simulink model "model"  (R2024b)
settings: Solver=ode4  StartTime=0.0  StopTime=tf  FixedStep=dt  RelTol=1e-3
values from neighbouring files (symbols this model uses):
  Controls_Matrix = [0,    XDE,   XDTH,      0 ... (first row only)    [aircraft_data_reader.m]
  dA = controls(1)    [compare_nonlinear_linear_approximate_simulator.m]
  dE = controls(2)    [compare_nonlinear_linear_approximate_simulator.m]
  dR = controls(4)    [compare_nonlinear_linear_approximate_simulator.m]
  dTH = controls(3)    [compare_nonlinear_linear_approximate_simulator.m]
  g = aircraft_data(52)    [aircraft_data_reader.m]
  Ixx = aircraft_data(53)    [aircraft_data_reader.m]
  Iyy = aircraft_data(54)    [aircraft_data_reader.m]
  Izz = aircraft_data(55)    [aircraft_data_reader.m]
  m = aircraft_data(51)    [aircraft_data_reader.m]
  mg0 = m*g * [ sin(s0(8)) ; -cos(s0(8))*sin(s0(7)) ; -cos(s0(8))*cos(s0(7)) ]    [aircraft_data_reader.m]
  p = states(4)    [Fdot.m]
  phi = states(7)    [Fdot.m]
  psi = states(9)    [Fdot.m]
  q = states(5)    [Fdot.m]
  r = states(6)    [Fdot.m]
  s0 = aircraft_data(4:15)    [aircraft_data_reader.m]
  States_Matrix = [Xu,   0,   Xw,    0,   0,   0,    0 ... (first row only)    [aircraft_data_reader.m]
  theta = states(8)    [Fdot.m]
  v = states(2)    [Fdot.m]
  w = states(3)    [Fdot.m]
  wdot = K4(3)    [RK4.m]
  x = states(10)    [Fdot.m]
  y = states(11)    [Fdot.m]
  z = states(12)    [Fdot.m]
undefined symbols (not defined in the file or in its folder): alpha, beta, d_a, d_e, d_r, d_th, initial_states_bus
libraries: simulink_extras x8, dspsigops x3, shared6dof x1, aerolibasang x1
settings Model: Creator=ahmed  LastModifiedBy=ahmed
settings DebuggingCC: SignalInfNanChecking=warning  CheckMatrixSingularityMsg=warning  SignalLabelMismatchMsg=warning  StateNameClashWarn=warning

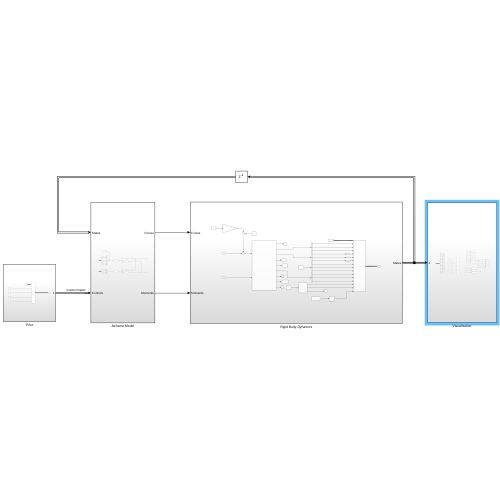
[thumbnail: Simulink's stored preview of the top-level diagram]
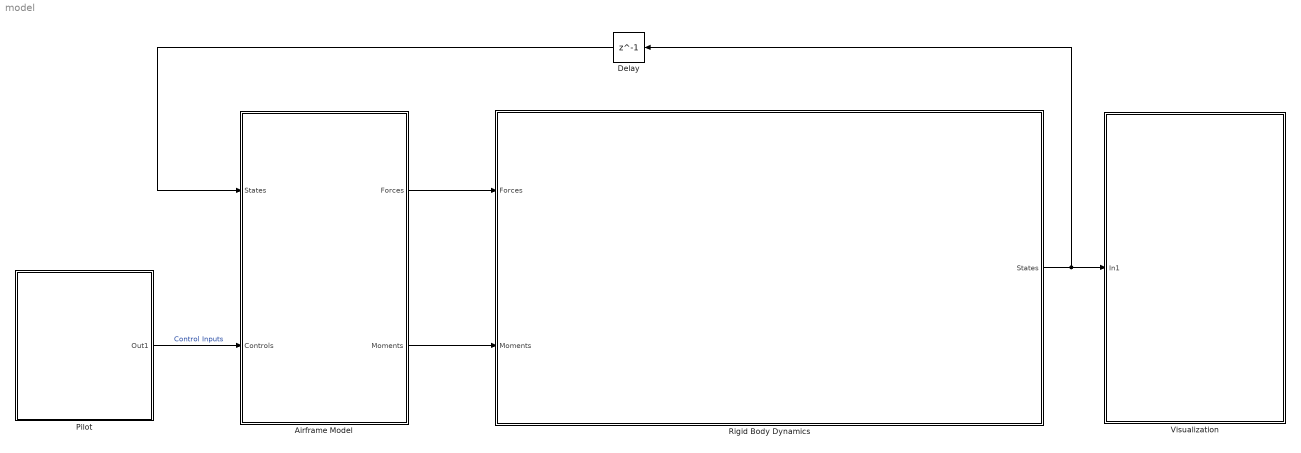
== system model ==
  Airframe Model : Subsystem
  Delay : Delay  DelayLength=1  InitialCondition=initial_states_bus
  Pilot : Subsystem
  Rigid Body Dynamics : Subsystem
  Visualization : Subsystem
  wires:
  Pilot/1(Out1) -> Airframe Model/2(Controls)  "Control Inputs"
  Airframe Model/1(Forces) -> Rigid Body Dynamics/1(Forces)
  Airframe Model/2(Moments) -> Rigid Body Dynamics/2(Moments)
  Rigid Body Dynamics/1(States) -> Visualization/1(In1), Delay/1
  Delay/1 -> Airframe Model/1(States)

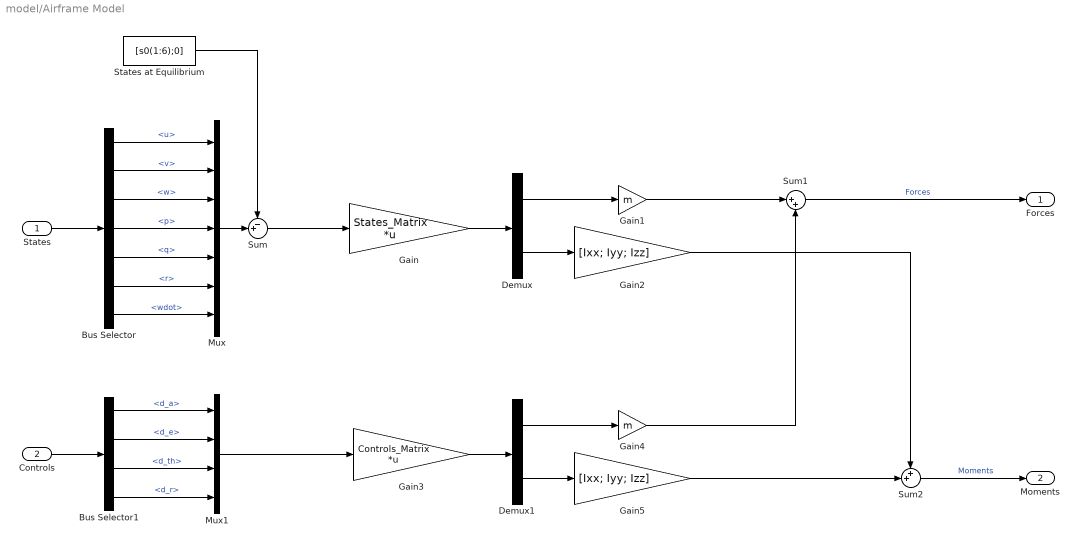
== system model/Airframe Model ==
  States : Inport  OutDataTypeStr=Bus: States_bus_T
  Controls : Inport  Port=2  OutDataTypeStr=Bus: Controls_bus_T
  Bus Selector : BusSelector  OutputSignals=u,v,w,p,q,r,wdot
  Bus Selector1 : BusSelector  OutputSignals=d_a,d_e,d_th,d_r
  Demux : Demux  Outputs=2
  Demux1 : Demux  Outputs=2
  Gain : Gain  Gain=States_Matrix  Multiplication=Matrix(K*u)
  Gain1 : Gain  Gain=m
  Gain2 : Gain  Gain=[Ixx; Iyy; Izz]
  Gain3 : Gain  Gain=Controls_Matrix  Multiplication=Matrix(K*u)
  Gain4 : Gain  Gain=m
  Gain5 : Gain  Gain=[Ixx; Iyy; Izz]
  Mux : Mux  Inputs=7
  Mux1 : Mux
  States at Equilibrium : Constant  Value=[s0(1:6);0]
  Sum : Sum  Inputs=-+|
  Sum1 : Sum  Inputs=|++
  Sum2 : Sum  Inputs=++|
  Forces : Outport
  Moments : Outport  Port=2
  wires:
  Sum1/1 -> Forces/1  "Forces"
  Sum2/1 -> Moments/1  "Moments"
  States/1 -> Bus Selector/1
  Bus Selector/2 -> Mux/2  "<v>"
  Bus Selector/1 -> Mux/1  "<u>"
  Bus Selector/3 -> Mux/3  "<w>"
  Bus Selector/4 -> Mux/4  "<p>"
  Bus Selector/5 -> Mux/5  "<q>"
  Bus Selector/6 -> Mux/6  "<r>"
  Bus Selector/7 -> Mux/7  "<wdot>"
  Mux/1 -> Sum/2
  States at Equilibrium/1 -> Sum/1
  Sum/1 -> Gain/1
  Gain/1 -> Demux/1
  Demux/1 -> Gain1/1
  Demux/2 -> Gain2/1
  Gain1/1 -> Sum1/1
  Gain2/1 -> Sum2/1
  Demux1/2 -> Gain5/1
  Gain3/1 -> Demux1/1
  Controls/1 -> Bus Selector1/1
  Bus Selector1/3 -> Mux1/3  "<d_th>"
  Bus Selector1/2 -> Mux1/2  "<d_e>"
  Bus Selector1/1 -> Mux1/1  "<d_a>"
  Bus Selector1/4 -> Mux1/4  "<d_r>"
  Mux1/1 -> Gain3/1
  Gain5/1 -> Sum2/2
  Demux1/1 -> Gain4/1
  Gain4/1 -> Sum1/2

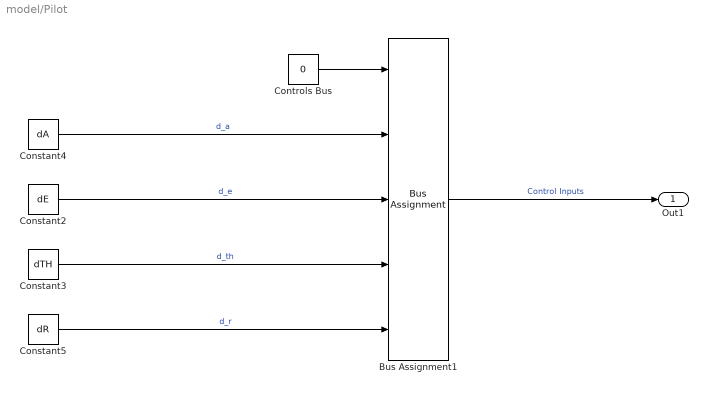
== system model/Pilot ==
  Bus Assignment1 : BusAssignment  AssignedSignals=d_a,d_e,d_th,d_r
  Constant2 : Constant  Value=dE
  Constant3 : Constant  Value=dTH
  Constant4 : Constant  Value=dA
  Constant5 : Constant  Value=dR
  Controls Bus : Constant  Value=0  OutDataTypeStr=Bus: Controls_bus_T
  Out1 : Outport
  wires:
  Constant2/1 -> Bus Assignment1/3  "d_e"
  Constant4/1 -> Bus Assignment1/2  "d_a"
  Constant5/1 -> Bus Assignment1/5  "d_r"
  Constant3/1 -> Bus Assignment1/4  "d_th"
  Controls Bus/1 -> Bus Assignment1/1
  Bus Assignment1/1 -> Out1/1  "Control Inputs"

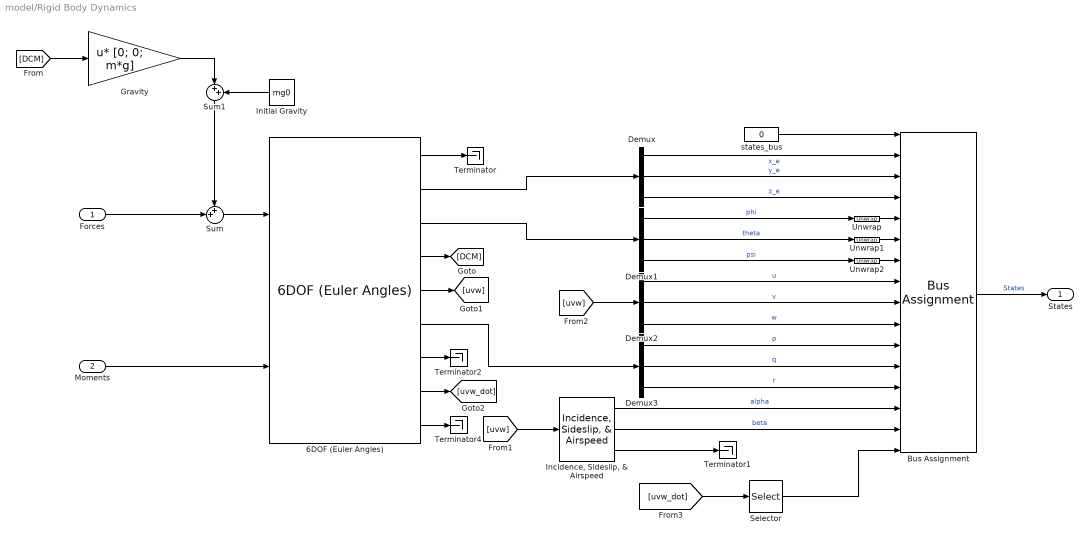
== system model/Rigid Body Dynamics ==
  Forces : Inport
  Moments : Inport  Port=2
  6DOF (Euler Angles) : shared6dof/6DOF (Euler Angles)  units=English (Velocity in ft/s)  mtype=Fixed  rep=Euler Angles  xme_0=s0(10:12)  Vm_0=s0(1:3)  eul_0=s0(7:9)  pm_0=s0(4:6)  mass_0=m  mass_e=0.5  mass_f=2.0  inertia=I  inertia_e=eye(3)  inertia_f=2*eye(3)  k_quat=1.0  vre_flag=on  abi_flag=on  aMode=0  xme_statename=''  Vm_statename=''  eul_statename=''  quat_statename=''  pm_statename=''  mass_statename=''
  Bus Assignment : BusAssignment  AssignedSignals=x,y,z,phi,theta,psi,u,v,w,p,q,r,alpha,beta,wdot
  Demux{,1..3} (4 alike) : Demux  Outputs=3
  Gravity : Gain  Gain=[0; 0; m*g]  Multiplication=Matrix(u*K)
  "Incidence, Sideslip, & Airspeed" : aerolibasang/Incidence, Sideslip, & Airspeed
  Initial Gravity : Constant  Value=mg0
  Selector : Selector  InputPortWidth=3  IndexOptions=Index vector (dialog)  Indices=3  OutputSizes=1
  Sum : Sum  Inputs=++|
  Sum1 : Sum  Inputs=|++
  Terminator{,1..2,4} (4 alike) : Terminator
  Unwrap : dspsigops/Unwrap  tol=pi  running=off
  Unwrap1 : dspsigops/Unwrap  tol=pi  running=off
  Unwrap2 : dspsigops/Unwrap  tol=pi  running=off
  states_bus : Constant  Value=0  OutDataTypeStr=Bus: States_bus_T
  States : Outport  OutDataTypeStr=Bus: States_bus_T
  wires:
  Bus Assignment/1 -> States/1  "States"
  Demux1/2 -> Unwrap1/1  "theta"
  Demux3/2 -> Bus Assignment/12  "q"
  6DOF (Euler Angles)/7 -> Terminator2/1
  6DOF (Euler Angles)/1 -> Terminator/1
  6DOF (Euler Angles)/3 -> Demux1/1
  states_bus/1 -> Bus Assignment/1
  Forces/1 -> Sum/2
  6DOF (Euler Angles)/6 -> Demux3/1
  6DOF (Euler Angles)/8 -> [uvw_dot]
  Demux2/2 -> Bus Assignment/9  "v"
  Demux1/3 -> Unwrap2/1  "psi"
  Demux3/3 -> Bus Assignment/13  "r"
  Demux2/1 -> Bus Assignment/8  "u"
  Demux2/3 -> Bus Assignment/10  "w"
  6DOF (Euler Angles)/2 -> Demux/1
  Demux/3 -> Bus Assignment/4  "z_e"
  Demux1/1 -> Unwrap/1  "phi"
  Demux/2 -> Bus Assignment/3  "y_e"
  Demux/1 -> Bus Assignment/2  "x_e"
  6DOF (Euler Angles)/9 -> Terminator4/1
  Demux3/1 -> Bus Assignment/11  "p"
  6DOF (Euler Angles)/4 -> [DCM]
  Unwrap/1 -> Bus Assignment/5
  Unwrap1/1 -> Bus Assignment/6
  Unwrap2/1 -> Bus Assignment/7
  [DCM] -> Gravity/1
  Gravity/1 -> Sum1/1
  Initial Gravity/1 -> Sum1/2
  Sum1/1 -> Sum/1
  Sum/1 -> 6DOF (Euler Angles)/1
  6DOF (Euler Angles)/5 -> [uvw]
  [uvw] -> "Incidence, Sideslip, & Airspeed"/1
  "Incidence, Sideslip, & Airspeed"/3 -> Terminator1/1
  "Incidence, Sideslip, & Airspeed"/2 -> Bus Assignment/15  "beta"
  "Incidence, Sideslip, & Airspeed"/1 -> Bus Assignment/14  "alpha"
  [uvw] -> Demux2/1
  Moments/1 -> 6DOF (Euler Angles)/2
  [uvw_dot] -> Selector/1
  Selector/1 -> Bus Assignment/16

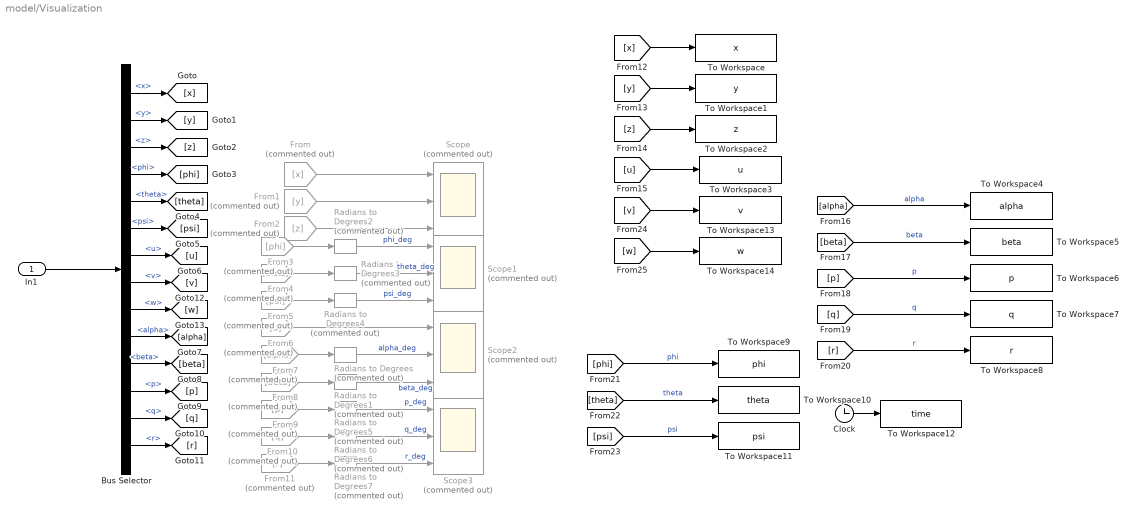
== system model/Visualization ==
  In1 : Inport
  Bus Selector : BusSelector  OutputSignals=x,y,z,phi,theta,psi,u,v,w,alpha,beta,p,q,r
  Clock : Clock
  From : From  Commented=on  GotoTag=x
  From1 : From  Commented=on  GotoTag=y
  From10 : From  Commented=on  GotoTag=q
  From11 : From  Commented=on  GotoTag=r
  From2 : From  Commented=on  GotoTag=z
  From3 : From  Commented=on  GotoTag=phi
  From4 : From  Commented=on  GotoTag=theta
  From5 : From  Commented=on  GotoTag=psi
  From6 : From  Commented=on  GotoTag=u
  From7 : From  Commented=on  GotoTag=alpha
  From8 : From  Commented=on  GotoTag=beta
  From9 : From  Commented=on  GotoTag=p
  Radians to Degrees{,1..7} (8 alike) : simulink_extras/Transformations/Radians to Degrees  Commented=on
  Scope{,1..3} (4 alike) : Scope  Commented=on  NumInputPorts=3
  To Workspace : ToWorkspace  VariableName=x  SaveFormat=Timeseries  SampleTime=-1
  To Workspace1 : ToWorkspace  VariableName=y  SaveFormat=Timeseries  SampleTime=-1
  To Workspace10 : ToWorkspace  VariableName=theta  SaveFormat=Timeseries  SampleTime=-1
  To Workspace11 : ToWorkspace  VariableName=psi  SaveFormat=Timeseries  SampleTime=-1
  To Workspace12 : ToWorkspace  VariableName=time  SaveFormat=Timeseries  SampleTime=-1
  To Workspace13 : ToWorkspace  VariableName=v  SaveFormat=Timeseries  SampleTime=-1
  To Workspace14 : ToWorkspace  VariableName=w  SaveFormat=Timeseries  SampleTime=-1
  To Workspace2 : ToWorkspace  VariableName=z  SaveFormat=Timeseries  SampleTime=-1
  To Workspace3 : ToWorkspace  VariableName=u  SaveFormat=Timeseries  SampleTime=-1
  To Workspace4 : ToWorkspace  VariableName=alpha  SaveFormat=Timeseries  SampleTime=-1
  To Workspace5 : ToWorkspace  VariableName=beta  SaveFormat=Timeseries  SampleTime=-1
  To Workspace6 : ToWorkspace  VariableName=p  SaveFormat=Timeseries  SampleTime=-1
  To Workspace7 : ToWorkspace  VariableName=q  SaveFormat=Timeseries  SampleTime=-1
  To Workspace8 : ToWorkspace  VariableName=r  SaveFormat=Timeseries  SampleTime=-1
  To Workspace9 : ToWorkspace  VariableName=phi  SaveFormat=Timeseries  SampleTime=-1
  wires:
  Bus Selector/6 -> [psi]  "<psi>"
  Bus Selector/1 -> [x]  "<x>"
  Bus Selector/7 -> [u]  "<u>"
  Bus Selector/4 -> [phi]  "<phi>"
  Bus Selector/10 -> [alpha]  "<alpha>"
  Bus Selector/14 -> [r]  "<r>"
  Bus Selector/11 -> [beta]  "<beta>"
  Bus Selector/5 -> [theta]  "<theta>"
  Bus Selector/13 -> [q]  "<q>"
  Bus Selector/12 -> [p]  "<p>"
  Bus Selector/2 -> [y]  "<y>"
  Bus Selector/3 -> [z]  "<z>"
  In1/1 -> Bus Selector/1
  Radians to Degrees/1 -> Scope2/2  "alpha_deg"
  Radians to Degrees1/1 -> Scope2/3  "beta_deg"
  Radians to Degrees2/1 -> Scope1/1  "phi_deg"
  Radians to Degrees3/1 -> Scope1/2  "theta_deg"
  Radians to Degrees4/1 -> Scope1/3  "psi_deg"
  From/1 -> Scope/1
  From1/1 -> Scope/2
  From2/1 -> Scope/3
  From3/1 -> Radians to Degrees2/1
  From4/1 -> Radians to Degrees3/1
  From5/1 -> Radians to Degrees4/1
  From6/1 -> Scope2/1
  From7/1 -> Radians to Degrees/1
  From8/1 -> Radians to Degrees1/1
  From9/1 -> Radians to Degrees5/1
  From10/1 -> Radians to Degrees6/1
  From11/1 -> Radians to Degrees7/1
  [x] -> To Workspace/1
  [y] -> To Workspace1/1
  [z] -> To Workspace2/1
  [u] -> To Workspace3/1
  Clock/1 -> To Workspace12/1
  Radians to Degrees5/1 -> Scope3/1  "p_deg"
  Radians to Degrees6/1 -> Scope3/2  "q_deg"
  Radians to Degrees7/1 -> Scope3/3  "r_deg"
  [phi] -> To Workspace9/1  "phi"
  [theta] -> To Workspace10/1  "theta"
  [psi] -> To Workspace11/1  "psi"
  [alpha] -> To Workspace4/1  "alpha"
  [beta] -> To Workspace5/1  "beta"
  [p] -> To Workspace6/1  "p"
  [q] -> To Workspace7/1  "q"
  [r] -> To Workspace8/1  "r"
  [v] -> To Workspace13/1
  Bus Selector/8 -> [v]  "<v>"
  Bus Selector/9 -> [w]  "<w>"
  [w] -> To Workspace14/1
